simulink model "AcermanDynExt"  (R2021a)
settings: Solver=FixedStepAuto  StartTime=0.0  StopTime=simTime  RelTol=1e-3
values from neighbouring files (symbols this model uses):
  a = 2    [Ackerman_init.m]
  a0 = 1    [Ackerman_init.m]
  a1 = 4    [Ackerman_init.m]
  a2 = 3    [Ackerman_init.m]
  b = 1.05*a    (= 2.1)    [Ackerman_init.m]
  Change = 0    [Ackerman_init.m]
  k0 = 1    [Ackerman_init.m]
  k1 = place(Ad,bd,pd)    [Ackerman_init.m]
  k2 = place(Ac,bc,lambdatr')    [Ackerman_init.m]
  l = ylabel('$\omega(t)$' )    [Ackerman_init.m]
  pathType = 1    [Ackerman_init.m]
  phi0 = 0    [Ackerman_init.m]
  r = 2    [Ackerman_init.m]
  ref0 = [0 0]'    [Ackerman_init.m]
  refType = 1    [Ackerman_init.m]
  T = 0.1    [Ackerman_init.m]
  theta0 = pi/2    (= 1.57079632679)    [Ackerman_init.m]
  v0 = 1    [Ackerman_init.m]
  v_ref = 2    [Ackerman_init.m]
  x0 = 1    [Ackerman_init.m]
  y0 = 1    [Ackerman_init.m]
libraries: robotmobilelib x5
(part 1 of 4)
settings Model: Creator=mohd-  LastModifiedBy=mebbaid
settings SolverCC: AlgebraicLoopSolver=TrustRegion
settings DebuggingCC: SFMachineParentedDataDiag=warning

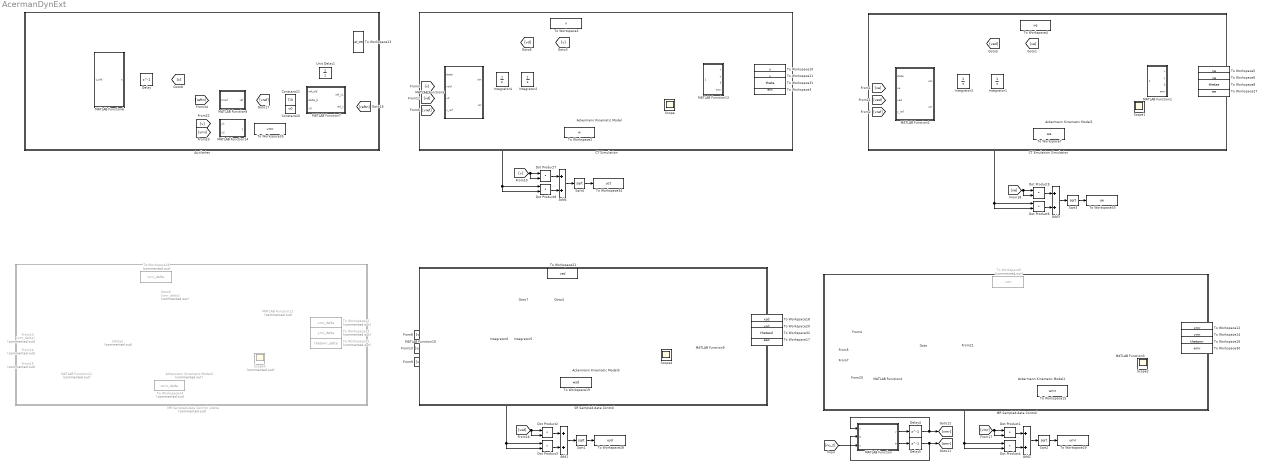
== system AcermanDynExt ==
  Ackermann Kinematic Model{,1..3} (4 alike) : robotmobilelib/Ackermann Kinematic Model  WheelBase=l  VehicleSpeedRange=[-inf inf]  MaxSteeringAngle=pi/3  InitialState=[x0; y0; theta0; phi0]  SimulateUsing=Interpreted execution
      settings: SourceProductBaseCode=RO
  Ackermann Kinematic Model4 : robotmobilelib/Ackermann Kinematic Model  Commented=on  WheelBase=l  VehicleSpeedRange=[-inf inf]  MaxSteeringAngle=pi/3  InitialState=[x0; y0; theta0; phi0]  SimulateUsing=Interpreted execution
      settings: SourceProductBaseCode=RO
  Add{1..4} (4 alike) : Sum
  Auxilaries : Subsystem
  CT Emulation Simulation : Subsystem
  CT Simulation : Subsystem
  Constant20 : Constant  Value=v0
  Constant21 : Constant  Value=T/3
  Delay : Delay  DelayLength=1  InitialCondition=0  SampleTime=T
  Delay2 : Delay  Commented=on  DelayLength=1  InitialCondition=v0  SampleTime=T
  Delay4 : Delay  DelayLength=1  InitialCondition=v0  SampleTime=T
  Delay5 : Delay  DelayLength=1  InitialCondition=0  SampleTime=T
  Dot Product{1..8} (8 alike) : DotProduct  InputSameDT=on  OutDataTypeStr=Inherit: Inherit via internal rule
  From10 : From  Commented=on  GotoTag=vmr_delta
  From14 : From  Commented=on  GotoTag=vref
  From15 : From  Commented=on  GotoTag=c
  Goto9 : Goto  Commented=on  GotoTag=vmr_delta
  Integrator1 : Integrator  InitialCondition=v0
  Integrator2 : Integrator  InitialCondition=v0
  Integrator3 : Integrator
  Integrator4 : Integrator
  Integrator5 : Integrator  InitialCondition=v0
  Integrator6 : Integrator
  MATLAB Function : MATLAB Function  TreatAsAtomicUnit=on  SystemSampleTime=T
  MATLAB Function1 : MATLAB Function  TreatAsAtomicUnit=on
  MATLAB Function10 : MATLAB Function  TreatAsAtomicUnit=on  SystemSampleTime=T
  MATLAB Function11 : MATLAB Function  Commented=on  TreatAsAtomicUnit=on
  MATLAB Function12 : MATLAB Function  Commented=on  TreatAsAtomicUnit=on  SystemSampleTime=T
  MATLAB Function13 : MATLAB Function  TreatAsAtomicUnit=on
  MATLAB Function14 : MATLAB Function  TreatAsAtomicUnit=on  SystemSampleTime=T
  MATLAB Function2 : MATLAB Function  TreatAsAtomicUnit=on  SystemSampleTime=T
  MATLAB Function3 : MATLAB Function  TreatAsAtomicUnit=on
  MATLAB Function4 : MATLAB Function  TreatAsAtomicUnit=on  SystemSampleTime=T/3
  MATLAB Function5 : MATLAB Function  TreatAsAtomicUnit=on
  MATLAB Function6 : MATLAB Function  TreatAsAtomicUnit=on  SystemSampleTime=T/3
  MATLAB Function7 : MATLAB Function  TreatAsAtomicUnit=on  SystemSampleTime=T
  MATLAB Function8 : MATLAB Function  TreatAsAtomicUnit=on
  MATLAB Function9 : MATLAB Function  TreatAsAtomicUnit=on
  MR Sampled-data Control : Subsystem
  MR Sampled-data Control ydelta : Subsystem  Commented=on
  SR Sampled-data Control : Subsystem
  Scope{,1..2,4} (4 alike) : Scope
  Scope3 : Scope  Commented=on
  Sqrt{1..4} (4 alike) : Sqrt  SaturateOnIntegerOverflow=on
  To Workspace1 : ToWorkspace  VariableName=v  SampleTime=10^-3
      settings: Save2DSignal=2-D array (concatenate along first dimension)
  To Workspace10 : ToWorkspace  VariableName=x  SampleTime=10^-3
      settings: Save2DSignal=2-D array (concatenate along first dimension)
  To Workspace11 : ToWorkspace  VariableName=y  SampleTime=10^-3
      settings: Save2DSignal=2-D array (concatenate along first dimension)
  To Workspace12 : ToWorkspace  VariableName=xmr  SampleTime=10^-3
      settings: Save2DSignal=2-D array (concatenate along first dimension)
  To Workspace13 : ToWorkspace  VariableName=ref_MR  SampleTime=T/3
  To Workspace14 : ToWorkspace  VariableName=ymr  SampleTime=10^-3
      settings: Save2DSignal=2-D array (concatenate along first dimension)
  To Workspace15 : ToWorkspace  VariableName=wmr  SampleTime=10^-3
      settings: Save2DSignal=2-D array (concatenate along first dimension)
  To Workspace16 : ToWorkspace  VariableName=thetamr  SampleTime=10^-3
      settings: Save2DSignal=2-D array (concatenate along first dimension)
  To Workspace17 : ToWorkspace  VariableName=esd  SampleTime=10^-3
      settings: Save2DSignal=2-D array (concatenate along first dimension)
  To Workspace18 : ToWorkspace  VariableName=xsd  SampleTime=10^-3
      settings: Save2DSignal=2-D array (concatenate along first dimension)
  To Workspace19 : ToWorkspace  VariableName=wsd  SampleTime=10^-3
      settings: Save2DSignal=2-D array (concatenate along first dimension)
  To Workspace2 : ToWorkspace  VariableName=w  SampleTime=10^-3
      settings: Save2DSignal=2-D array (concatenate along first dimension)
  To Workspace20 : ToWorkspace  VariableName=ysd  SampleTime=10^-3
      settings: Save2DSignal=2-D array (concatenate along first dimension)
  To Workspace21 : ToWorkspace  VariableName=vsd  SampleTime=10^-3
      settings: Save2DSignal=2-D array (concatenate along first dimension)
  To Workspace22 : ToWorkspace  Commented=on  VariableName=xmr_delta  SampleTime=10^-3
      settings: Save2DSignal=2-D array (concatenate along first dimension)
  To Workspace23 : ToWorkspace  Commented=on  VariableName=ymr_delta  SampleTime=10^-3
      settings: Save2DSignal=2-D array (concatenate along first dimension)
  To Workspace24 : ToWorkspace  Commented=on  VariableName=wmr_delta  SampleTime=10^-3
      settings: Save2DSignal=2-D array (concatenate along first dimension)
  To Workspace25 : ToWorkspace  Commented=on  VariableName=thetamr_delta  SampleTime=10^-3
      settings: Save2DSignal=2-D array (concatenate along first dimension)
  To Workspace26 : ToWorkspace  Commented=on  VariableName=vmr_delta  SampleTime=10^-3
      settings: Save2DSignal=2-D array (concatenate along first dimension)
  To Workspace27 : ToWorkspace  VariableName=ee  SampleTime=10^-3
      settings: Save2DSignal=2-D array (concatenate along first dimension)
  To Workspace28 : ToWorkspace  VariableName=usd  SampleTime=10^-3
      settings: Save2DSignal=2-D array (concatenate along first dimension)
  To Workspace29 : ToWorkspace  VariableName=umr  SampleTime=10^-3
      settings: Save2DSignal=2-D array (concatenate along first dimension)
  To Workspace3 : ToWorkspace  VariableName=ect  SampleTime=10^-3
      settings: Save2DSignal=2-D array (concatenate along first dimension)
  To Workspace30 : ToWorkspace  VariableName=emr  SampleTime=10^-3
      settings: Save2DSignal=2-D array (concatenate along first dimension)
  To Workspace31 : ToWorkspace  VariableName=theta  SampleTime=10^-3
      settings: Save2DSignal=2-D array (concatenate along first dimension)
  To Workspace32 : ToWorkspace  VariableName=thetasd  SampleTime=10^-3
      settings: Save2DSignal=2-D array (concatenate along first dimension)
  To Workspace33 : ToWorkspace  VariableName=ue  SampleTime=10^-3
      settings: Save2DSignal=2-D array (concatenate along first dimension)
  To Workspace34 : ToWorkspace  VariableName=uct  SampleTime=10^-3
      settings: Save2DSignal=2-D array (concatenate along first dimension)
  To Workspace35 : ToWorkspace  VariableName=vmr  SampleTime=10^-3
      settings: Save2DSignal=2-D array (concatenate along first dimension)
  To Workspace4 : ToWorkspace  VariableName=ve  SampleTime=10^-3
      settings: Save2DSignal=2-D array (concatenate along first dimension)
  To Workspace5 : ToWorkspace  VariableName=xe  SampleTime=10^-3
      settings: Save2DSignal=2-D array (concatenate along first dimension)
  To Workspace6 : ToWorkspace  VariableName=ye  SampleTime=10^-3
      settings: Save2DSignal=2-D array (concatenate along first dimension)
  To Workspace7 : ToWorkspace  VariableName=we  SampleTime=10^-3
      settings: Save2DSignal=2-D array (concatenate along first dimension)
  To Workspace8 : ToWorkspace  VariableName=thetae  SampleTime=10^-3
      settings: Save2DSignal=2-D array (concatenate along first dimension)
  To Workspace9 : ToWorkspace  Commented=on  VariableName=vmr  SampleTime=10^-3
      settings: Save2DSignal=2-D array (concatenate along first dimension)
  Unit Delay1 : UnitDelay  InitialCondition=ref0  SampleTime=T/3  HasFrameUpgradeWarning=on
  wires:
  Ackermann Kinematic Model3/2 -> Scope4/1
  Ackermann Kinematic Model2/1 -> MATLAB Function4/1(state), MATLAB Function3/1(state)
  [vmr] -> MATLAB Function4/2(v)
  Constant20/1 -> MATLAB Function7/3(v0)
  Ackermann Kinematic Model2/2 -> Scope2/1
  MATLAB Function1/1(x) -> To Workspace5/1
  Delay/1 -> [c], MATLAB Function6/1(c_old)
  MATLAB Function1/3(theta) -> To Workspace8/1
  MATLAB Function10/2(utr) -> Dot Product3/2, Dot Product3/1, To Workspace19/1, Ackermann Kinematic Model3/2
  MATLAB Function5/1(utn) -> Integrator4/1
  [vref] -> MATLAB Function10/4(v_ref)
  MATLAB Function6/1(c) -> Delay/1
  [c] -> MATLAB Function4/4(c)
  MATLAB Function8/1(ref) -> [vref]
  [v] -> MATLAB Function5/2(vold)
  Ackermann Kinematic Model/2 -> Scope/1
  [vref] -> MATLAB Function5/4(v_ref)
  MATLAB Function2/1(utn) -> Integrator3/1
  Integrator2/1 -> To Workspace1/1, [v], Ackermann Kinematic Model/1
  [ve] -> MATLAB Function2/2(ve)
  Ackermann Kinematic Model1/2 -> Scope1/1
  MATLAB Function7/1(ref_x1) -> To Workspace13/1, Unit Delay1/1
  [vref] -> MATLAB Function2/4(v_ref)
  Ackermann Kinematic Model1/1 -> MATLAB Function2/1(state), MATLAB Function1/1(state)
  MATLAB Function1/2(y) -> To Workspace6/1
  [vsd] -> MATLAB Function10/2(v)
  MATLAB Function7/2(ref_x) -> [reftn]
  [vref] -> MATLAB Function4/3(v_ref)
  [reftn] -> MATLAB Function8/1(tnref)
  Integrator1/1 -> To Workspace4/1, [ve], Ackermann Kinematic Model1/1
  Constant21/1 -> MATLAB Function7/2(delta_b)
  MATLAB Function10/1(utn) -> Integrator6/1
  Integrator5/1 -> To Workspace21/1, [vsd], Ackermann Kinematic Model3/1
  Unit Delay1/1 -> MATLAB Function7/1(ref_old)
  Integrator3/1 -> [ved], Integrator1/1
  [ved] -> MATLAB Function2/3(ved)
  Integrator4/1 -> [vd], Integrator2/1
  [vd] -> MATLAB Function5/3(vd)
  Integrator6/1 -> [vsdd], Integrator5/1
  [vsdd] -> MATLAB Function10/3(vsdd)
  MATLAB Function11/1(x) -> To Workspace22/1
  MATLAB Function12/2(w) -> To Workspace24/1, Ackermann Kinematic Model4/2
  MATLAB Function11/2(y) -> To Workspace23/1
  Ackermann Kinematic Model4/2 -> Scope3/1
  Delay2/1 -> To Workspace26/1, Goto9/1, Ackermann Kinematic Model4/1
  From14/1 -> MATLAB Function12/3(v_ref)
  MATLAB Function12/1(u) -> Delay2/1
  From15/1 -> MATLAB Function12/4(c)
  MATLAB Function11/3(theta) -> To Workspace25/1
  Ackermann Kinematic Model4/1 -> MATLAB Function12/1(state), MATLAB Function11/1(state)
  From10/1 -> MATLAB Function12/2(v)
  MATLAB Function3/2(y) -> To Workspace14/1
  MATLAB Function3/1(x) -> To Workspace12/1
  MATLAB Function3/3(theta) -> To Workspace16/1
  MATLAB Function3/4(emr) -> To Workspace30/1
  MATLAB Function1/4(emr) -> To Workspace27/1
  Ackermann Kinematic Model/1 -> MATLAB Function13/1(state), MATLAB Function5/1(state)
  MATLAB Function13/3(theta) -> To Workspace31/1
  MATLAB Function13/4(emr) -> To Workspace3/1
  MATLAB Function13/1(x) -> To Workspace10/1
  MATLAB Function13/2(y) -> To Workspace11/1
  Ackermann Kinematic Model3/1 -> MATLAB Function9/1(state), MATLAB Function10/1(state)
  MATLAB Function9/3(theta) -> To Workspace32/1
  MATLAB Function9/4(emr) -> To Workspace17/1
  MATLAB Function9/1(x) -> To Workspace18/1
  MATLAB Function9/2(y) -> To Workspace20/1
  Add1/1 -> Sqrt1/1
  Dot Product2/1 -> Add1/1
  Dot Product3/1 -> Add1/2
  Sqrt1/1 -> To Workspace28/1
  [vsd] -> Dot Product2/2, Dot Product2/1
  Dot Product1/1 -> Add2/1
  Dot Product4/1 -> Add2/2
  Sqrt2/1 -> To Workspace29/1
  Add2/1 -> Sqrt2/1
  MATLAB Function4/2(w) -> Dot Product4/1, Dot Product4/2, To Workspace15/1, Ackermann Kinematic Model2/2
  [vmr] -> Dot Product1/2, Dot Product1/1
  Dot Product5/1 -> Add3/1
  Dot Product6/1 -> Add3/2
  Sqrt3/1 -> To Workspace33/1
  Add3/1 -> Sqrt3/1
  MATLAB Function2/2(utr) -> Dot Product6/1, Dot Product6/2, To Workspace7/1, Ackermann Kinematic Model1/2
  [ve] -> Dot Product5/2, Dot Product5/1
  Dot Product7/1 -> Add4/1
  Dot Product8/1 -> Add4/2
  Sqrt4/1 -> To Workspace34/1
  Add4/1 -> Sqrt4/1
  MATLAB Function5/2(utr) -> Dot Product8/1, Dot Product8/2, To Workspace2/1, Ackermann Kinematic Model/2
  [v] -> Dot Product7/2, Dot Product7/1
  [vmr] -> To Workspace9/1, Ackermann Kinematic Model2/1
  [amr] -> MATLAB Function4/5(amr)
  MATLAB Function/1(v) -> Delay4/1
  MATLAB Function/2(a) -> Delay5/1
  Delay4/1 -> MATLAB Function/1("v "), [vmr]
  Delay5/1 -> [amr], MATLAB Function/2("a ")
  MATLAB Function4/1(u) -> [nu_2]
  [nu_2] -> MATLAB Function/3(u)
  [v] -> MATLAB Function14/1(u1)
  MATLAB Function14/1(y) -> To Workspace35/1
  [vmr] -> MATLAB Function14/2(u2)

== system AcermanDynExt/Auxilaries ==

== system AcermanDynExt/CT Emulation Simulation ==

== system AcermanDynExt/CT Simulation ==

== system AcermanDynExt/MR Sampled-data Control ==

== system AcermanDynExt/MR Sampled-data Control ydelta ==

== system AcermanDynExt/SR Sampled-data Control ==

== matlab function AcermanDynExt/MATLAB Function4 ==
  data: state input; v input; v_ref input; c input; amr input; pathType parameter; r parameter; a2 parameter; a1 parameter; a0 parameter; k0 parameter; l parameter; u output; w output; Change parameter; T parameter; refType parameter
function [u,w] = MATLAB_Function5(state, v, v_ref, c , amr,pathType, r, a2, a1, a0, k0, l , Change, T, refType)

x = state(1); y = state(2); z = state(3); theta = state(4);

d = T/3; 
if refType == 1
    lamda1 = k0; lamda2 = k0;
    L0 = -(exp(-T*lamda1) + exp(-T*lamda2) - exp(-T*lamda1)*exp(-T*lamda2) - 1)/T^2;
    L1 = -(exp(-T*lamda1) + exp(-T*lamda2) + exp(-T*lamda1)*exp(-T*lamda2) - 3)/(2*T);
else
    L0 = 0;
    L1 = 0;
end
 

if pathType == 1
    w0 = [   -(2*a2*l^2*v^2*cos(theta)^2 - 2*v^3*y*sin(z) - a0*l^2*r^2*cos(theta)^2 - 2*v^3*x*cos(z) + a0*l^2*x^2*cos(theta)^2 + a0*l^2*y^2*cos(theta)^2 + 2*v^3*x*cos(theta)^2*cos(z) + 2*v^3*y*cos(theta)^2*sin(z) + 2*a1*l^2*v*x*cos(theta)^2*cos(z) + 2*a1*l^2*v*y*cos(theta)^2*sin(z) + 2*a2*l*v^2*y*cos(theta)*cos(z)*sin(theta) - 2*a2*l*v^2*x*cos(theta)*sin(theta)*sin(z))/(2*l*v^2*(y*cos(z) - x*sin(z)));
             -(2*a2*l^2*v^2*cos(theta)^2 - 2*v^3*y*sin(z) - a0*l^2*r^2*cos(theta)^2 - 2*v^3*x*cos(z) + a0*l^2*x^2*cos(theta)^2 + a0*l^2*y^2*cos(theta)^2 + 2*v^3*x*cos(theta)^2*cos(z) + 2*v^3*y*cos(theta)^2*sin(z) + 2*a1*l^2*v*x*cos(theta)^2*cos(z) + 2*a1*l^2*v*y*cos(theta)^2*sin(z) + 2*a2*l*v^2*y*cos(theta)*cos(z)*sin(theta) - 2*a2*l*v^2*x*cos(theta)*sin(theta)*sin(z))/(2*l*v^2*(y*cos(z) - x*sin(z)));
             -(2*a2*l^2*v^2*cos(theta)^2 - 2*v^3*y*sin(z) - a0*l^2*r^2*cos(theta)^2 - 2*v^3*x*cos(z) + a0*l^2*x^2*cos(theta)^2 + a0*l^2*y^2*cos(theta)^2 + 2*v^3*x*cos(theta)^2*cos(z) + 2*v^3*y*cos(theta)^2*sin(z) + 2*a1*l^2*v*x*cos(theta)^2*cos(z) + 2*a1*l^2*v*y*cos(theta)^2*sin(z) + 2*a2*l*v^2*y*cos(theta)*cos(z)*sin(theta) - 2*a2*l*v^2*x*cos(theta)*sin(theta)*sin(z))/(2*l*v^2*(y*cos(z) - x*sin(z)))]; 
 
    w1 = [  -(3*(2*l*v^6*y*cos(theta)^3*cos(z) - 2*v^6*y^2*cos(z)^2*sin(theta) - 2*v^6*x^2*sin(theta)*sin(z)^2 - 2*v^6*y^2*sin(theta)*sin(z)^2 - 2*v^6*x^2*cos(z)^2*sin(theta) - 2*l*v^6*x*cos(theta)^3*sin(z) - 2*v^6*x^2*cos(theta)^2*cos(z)^2*sin(theta) + 4*v^6*x^2*cos(theta)^4*cos(z)^2*sin(theta) + 2*v^6*y^2*cos(theta)^2*cos(z)^2*sin(theta) + 2*v^6*x^2*cos(theta)^2*sin(theta)*sin(z)^2 - 2*v^6*y^2*cos(theta)^2*sin(theta)*sin(z)^2 + 4*v^6*y^2*cos(theta)^4*sin(theta)*sin(z)^2 - 2*l*v^6*y*cos(theta)*cos(z) + a0^2*l^4*r^4*cos(theta)^4*sin(theta) + 2*l*v^6*x*cos(theta)*sin(z) + 4*a2^2*l^4*v^4*cos(theta)^4*sin(theta) + a0^2*l^4*x^4*cos(theta)^4*sin(theta) + a0^2*l^4*y^4*cos(theta)^4*sin(theta) - 2*a2^2*l^3*v^4*y*cos(theta)^3*cos(z) + 2*a2^2*l^3*v^4*x*cos(theta)^3*sin(z) - 2*a0^2*l^4*r^2*x^2*cos(theta)^4*sin(theta) - 2*a0^2*l^4*r^2*y^2*cos(theta)^4*sin(theta) + 2*a0^2*l^4*x^2*y^2*cos(theta)^4*sin(theta) + 2*a1*l^3*v^4*y*cos(theta)^3*cos(z) - 2*a1*l^3*v^4*x*cos(theta)^3*sin(z) - 2*a2^2*l^2*v^4*x^2*cos(theta)^2*sin(theta)*sin(z)^2 + 4*a1^2*l^4*v^2*y^2*cos(theta)^4*sin(theta)*sin(z)^2 - 8*v^6*x*y*cos(theta)^2*cos(z)*sin(theta)*sin(z) + 8*v^6*x*y*cos(theta)^4*cos(z)*sin(theta)*sin(z) - a0*l^2*v^3*x^3*cos(theta)^2*cos(z)*sin(theta) + 4*a0*l^2*v^3*x^3*cos(theta)^4*cos(z)*sin(theta) - 2*a0*l^3*v^3*x^2*cos(theta)^3*cos(z)*sin(z) + 2*a0*l^3*v^3*y^2*cos(theta)^3*cos(z)*sin(z) - a0*l^2*v^3*y^3*cos(theta)^2*sin(theta)*sin(z) + 4*a0*l^2*v^3*y^3*cos(theta)^4*sin(theta)*sin(z) + 4*a2^2*l^2*v^4*y^2*cos(theta)^2*cos(z)^2*sin(theta)^3 + 4*a2^2*l^2*v^4*x^2*cos(theta)^2*sin(theta)^3*sin(z)^2 - 2*a1*l^2*v^4*x^2*cos(theta)^2*cos(z)^2*sin(theta) + 8*a1*l^2*v^4*x^2*cos(theta)^4*cos(z)^2*sin(theta) + 2*a1*l^2*v^4*y^2*cos(theta)^2*cos(z)^2*sin(theta) + 8*a2^2*l^3*v^4*y*cos(theta)^3*cos(z)*sin(theta)^2 + 2*a1*l^2*v^4*x^2*cos(theta)^2*sin(theta)*sin(z)^2 - 8*a2^2*l^3*v^4*x*cos(theta)^3*sin(theta)^2*sin(z) - 2*a1*l^2*v^4*y^2*cos(theta)^2*sin(theta)*sin(z)^2 + 8*a1*l^2*v^4*y^2*cos(theta)^4*sin(theta)*sin(z)^2 - a0*a2*l^3*v^2*y^3*cos(theta)^3*cos(z) - 4*a0*a2*l^4*r^2*v^2*cos(theta)^4*sin(theta) + 4*a0*a2*l^4*v^2*x^2*cos(theta)^4*sin(theta) + 4*a0*a2*l^4*v^2*y^2*cos(theta)^4*sin(theta) + a0*a2*l^3*v^2*x^3*cos(theta)^3*sin(z) + 2*a0*l^3*v^3*x*y*cos(theta)^3*cos(z)^2 - 2*a2*l^2*v^5*x*cos(theta)^2*cos(z)*sin(theta) + 8*a2*l^2*v^5*x*cos(theta)^4*cos(z)*sin(theta) - 2*a0*l^3*v^3*x*y*cos(theta)^3*sin(z)^2 - 2*a2*l^2*v^5*y*cos(theta)^2*sin(theta)*sin(z) + 8*a2*l^2*v^5*y*cos(theta)^4*sin(theta)*sin(z) + 4*a1^2*l^4*v^2*x^2*cos(theta)^4*cos(z)^2*sin(theta) - 2*a2^2*l^2*v^4*y^2*cos(theta)^2*cos(z)^2*sin(theta) - 4*a0*a2*l^3*v^2*x^3*cos(theta)^3*sin(theta)^2*sin(z) + a0*a2*l^3*r^2*v^2*y*cos(theta)^3*cos(z) - 8*a2*l*v^5*x^2*cos(theta)^3*cos(z)*sin(theta)^2*sin(z) + 8*a2*l*v^5*y^2*cos(theta)^3*cos(z)*sin(theta)^2*sin(z) - a0*a2*l^3*v^2*x^2*y*cos(theta)^3*cos(z) - 2*a1*a2*l^3*v^3*x*y*cos(theta)^3*cos(z)^2 - a0*a2*l^3*r^2*v^2*x*cos(theta)^3*sin(z) + 4*a0*a1*l^4*v*x^3*cos(theta)^4*cos(z)*sin(theta) + 8*a1*a2*l^4*v^3*x*cos(theta)^4*cos(z)*sin(theta) + a0*a2*l^3*v^2*x*y^2*cos(theta)^3*sin(z) + 2*a1*a2*l^3*v^3*x*y*cos(theta)^3*sin(z)^2 + 4*a0*a1*l^4*v*y^3*cos(theta)^4*sin(theta)*sin(z) + 8*a1*a2*l^4*v^3*y*cos(theta)^4*sin(theta)*sin(z) - 2*a2*l*v^5*x*y*cos(theta)*cos(z)^2*sin(theta)^2 + 2*a2*l*v^5*x*y*cos(theta)*sin(theta)^2*sin(z)^2 + 2*a1*a2*l^3*v^3*x^2*cos(theta)^3*cos(z)*sin(z) - 2*a1*a2*l^3*v^3*y^2*cos(theta)^3*cos(z)*sin(z) + a0*l^2*r^2*v^3*x*cos(theta)^2*cos(z)*sin(theta) - 4*a0*l^2*r^2*v^3*x*cos(theta)^4*cos(z)*sin(theta) - a0*l^2*v^3*x*y^2*cos(theta)^2*cos(z)*sin(theta) + 4*a0*l^2*v^3*x*y^2*cos(theta)^4*cos(z)*sin(theta) + 8*a2*l*v^5*x*y*cos(theta)^3*cos(z)^2*sin(theta)^2 + a0*l^2*r^2*v^3*y*cos(theta)^2*sin(theta)*sin(z) - 4*a0*l^2*r^2*v^3*y*cos(theta)^4*sin(theta)*sin(z) - a0*l^2*v^3*x^2*y*cos(theta)^2*sin(theta)*sin(z) + 4*a0*l^2*v^3*x^2*y*cos(theta)^4*sin(theta)*sin(z) - 8*a2*l*v^5*x*y*cos(theta)^3*sin(theta)^2*sin(z)^2 + 2*a2*l*v^5*x^2*cos(theta)*cos(z)*sin(theta)^2*sin(z) - 2*a2*l*v^5*y^2*cos(theta)*cos(z)*sin(theta)^2*sin(z) + 4*a0*a2*l^3*v^2*y^3*cos(theta)^3*cos(z)*sin(theta)^2 - 8*a1*l^2*v^4*x*y*cos(theta)^2*cos(z)*sin(theta)*sin(z) + 16*a1*l^2*v^4*x*y*cos(theta)^4*cos(z)*sin(theta)*sin(z) - 4*a0*a2*l^3*r^2*v^2*y*cos(theta)^3*cos(z)*sin(theta)^2 + 4*a0*a2*l^3*v^2*x^2*y*cos(theta)^3*cos(z)*sin(theta)^2 + 8*a1*a2*l^3*v^3*x*y*cos(theta)^3*cos(z)^2*sin(theta)^2 + 4*a0*a2*l^3*r^2*v^2*x*cos(theta)^3*sin(theta)^2*sin(z) - 4*a0*a2*l^3*v^2*x*y^2*cos(theta)^3*sin(theta)^2*sin(z) - 8*a1*a2*l^3*v^3*x*y*cos(theta)^3*sin(theta)^2*sin(z)^2 + 4*a2^2*l^2*v^4*x*y*cos(theta)^2*cos(z)*sin(theta)*sin(z) + 8*a1^2*l^4*v^2*x*y*cos(theta)^4*cos(z)*sin(theta)*sin(z) - 4*a0*a1*l^4*r^2*v*x*cos(theta)^4*cos(z)*sin(theta) + 4*a0*a1*l^4*v*x*y^2*cos(theta)^4*cos(z)*sin(theta) - 4*a0*a1*l^4*r^2*v*y*cos(theta)^4*sin(theta)*sin(z) + 4*a0*a1*l^4*v*x^2*y*cos(theta)^4*sin(theta)*sin(z) - 8*a1*a2*l^3*v^3*x^2*cos(theta)^3*cos(z)*sin(theta)^2*sin(z) + 8*a1*a2*l^3*v^3*y^2*cos(theta)^3*cos(z)*sin(theta)^2*sin(z) - 8*a2^2*l^2*v^4*x*y*cos(theta)^2*cos(z)*sin(theta)^3*sin(z)))/(8*l^2*v^4*cos(theta)*(y*cos(z) - x*sin(z))^2);
            -(3*(2*l*v^6*y*cos(theta)^3*cos(z) - 2*v^6*y^2*cos(z)^2*sin(theta) - 2*v^6*x^2*sin(theta)*sin(z)^2 - 2*v^6*y^2*sin(theta)*sin(z)^2 - 2*v^6*x^2*cos(z)^2*sin(theta) - 2*l*v^6*x*cos(theta)^3*sin(z) - 2*v^6*x^2*cos(theta)^2*cos(z)^2*sin(theta) + 4*v^6*x^2*cos(theta)^4*cos(z)^2*sin(theta) + 2*v^6*y^2*cos(theta)^2*cos(z)^2*sin(theta) + 2*v^6*x^2*cos(theta)^2*sin(theta)*sin(z)^2 - 2*v^6*y^2*cos(theta)^2*sin(theta)*sin(z)^2 + 4*v^6*y^2*cos(theta)^4*sin(theta)*sin(z)^2 - 2*l*v^6*y*cos(theta)*cos(z) + a0^2*l^4*r^4*cos(theta)^4*sin(theta) + 2*l*v^6*x*cos(theta)*sin(z) + 4*a2^2*l^4*v^4*cos(theta)^4*sin(theta) + a0^2*l^4*x^4*cos(theta)^4*sin(theta) + a0^2*l^4*y^4*cos(theta)^4*sin(theta) - 2*a2^2*l^3*v^4*y*cos(theta)^3*cos(z) + 2*a2^2*l^3*v^4*x*cos(theta)^3*sin(z) - 2*a0^2*l^4*r^2*x^2*cos(theta)^4*sin(theta) - 2*a0^2*l^4*r^2*y^2*cos(theta)^4*sin(theta) + 2*a0^2*l^4*x^2*y^2*cos(theta)^4*sin(theta) + 2*a1*l^3*v^4*y*cos(theta)^3*cos(z) - 2*a1*l^3*v^4*x*cos(theta)^3*sin(z) - 2*a2^2*l^2*v^4*x^2*cos(theta)^2*sin(theta)*sin(z)^2 + 4*a1^2*l^4*v^2*y^2*cos(theta)^4*sin(theta)*sin(z)^2 - 8*v^6*x*y*cos(theta)^2*cos(z)*sin(theta)*sin(z) + 8*v^6*x*y*cos(theta)^4*cos(z)*sin(theta)*sin(z) - a0*l^2*v^3*x^3*cos(theta)^2*cos(z)*sin(theta) + 4*a0*l^2*v^3*x^3*cos(theta)^4*cos(z)*sin(theta) - 2*a0*l^3*v^3*x^2*cos(theta)^3*cos(z)*sin(z) + 2*a0*l^3*v^3*y^2*cos(theta)^3*cos(z)*sin(z) - a0*l^2*v^3*y^3*cos(theta)^2*sin(theta)*sin(z) + 4*a0*l^2*v^3*y^3*cos(theta)^4*sin(theta)*sin(z) + 4*a2^2*l^2*v^4*y^2*cos(theta)^2*cos(z)^2*sin(theta)^3 + 4*a2^2*l^2*v^4*x^2*cos(theta)^2*sin(theta)^3*sin(z)^2 - 2*a1*l^2*v^4*x^2*cos(theta)^2*cos(z)^2*sin(theta) + 8*a1*l^2*v^4*x^2*cos(theta)^4*cos(z)^2*sin(theta) + 2*a1*l^2*v^4*y^2*cos(theta)^2*cos(z)^2*sin(theta) + 8*a2^2*l^3*v^4*y*cos(theta)^3*cos(z)*sin(theta)^2 + 2*a1*l^2*v^4*x^2*cos(theta)^2*sin(theta)*sin(z)^2 - 8*a2^2*l^3*v^4*x*cos(theta)^3*sin(theta)^2*sin(z) - 2*a1*l^2*v^4*y^2*cos(theta)^2*sin(theta)*sin(z)^2 + 8*a1*l^2*v^4*y^2*cos(theta)^4*sin(theta)*sin(z)^2 - a0*a2*l^3*v^2*y^3*cos(theta)^3*cos(z) - 4*a0*a2*l^4*r^2*v^2*cos(theta)^4*sin(theta) + 4*a0*a2*l^4*v^2*x^2*cos(theta)^4*sin(theta) + 4*a0*a2*l^4*v^2*y^2*cos(theta)^4*sin(theta) + a0*a2*l^3*v^2*x^3*cos(theta)^3*sin(z) + 2*a0*l^3*v^3*x*y*cos(theta)^3*cos(z)^2 - 2*a2*l^2*v^5*x*cos(theta)^2*cos(z)*sin(theta) + 8*a2*l^2*v^5*x*cos(theta)^4*cos(z)*sin(theta) - 2*a0*l^3*v^3*x*y*cos(theta)^3*sin(z)^2 - 2*a2*l^2*v^5*y*cos(theta)^2*sin(theta)*sin(z) + 8*a2*l^2*v^5*y*cos(theta)^4*sin(theta)*sin(z) + 4*a1^2*l^4*v^2*x^2*cos(theta)^4*cos(z)^2*sin(theta) - 2*a2^2*l^2*v^4*y^2*cos(theta)^2*cos(z)^2*sin(theta) - 4*a0*a2*l^3*v^2*x^3*cos(theta)^3*sin(theta)^2*sin(z) + a0*a2*l^3*r^2*v^2*y*cos(theta)^3*cos(z) - 8*a2*l*v^5*x^2*cos(theta)^3*cos(z)*sin(theta)^2*sin(z) + 8*a2*l*v^5*y^2*cos(theta)^3*cos(z)*sin(theta)^2*sin(z) - a0*a2*l^3*v^2*x^2*y*cos(theta)^3*cos(z) - 2*a1*a2*l^3*v^3*x*y*cos(theta)^3*cos(z)^2 - a0*a2*l^3*r^2*v^2*x*cos(theta)^3*sin(z) + 4*a0*a1*l^4*v*x^3*cos(theta)^4*cos(z)*sin(theta) + 8*a1*a2*l^4*v^3*x*cos(theta)^4*cos(z)*sin(theta) + a0*a2*l^3*v^2*x*y^2*cos(theta)^3*sin(z) + 2*a1*a2*l^3*v^3*x*y*cos(theta)^3*sin(z)^2 + 4*a0*a1*l^4*v*y^3*cos(theta)^4*sin(theta)*sin(z) + 8*a1*a2*l^4*v^3*y*cos(theta)^4*sin(theta)*sin(z) - 2*a2*l*v^5*x*y*cos(theta)*cos(z)^2*sin(theta)^2 + 2*a2*l*v^5*x*y*cos(theta)*sin(theta)^2*sin(z)^2 + 2*a1*a2*l^3*v^3*x^2*cos(theta)^3*cos(z)*sin(z) - 2*a1*a2*l^3*v^3*y^2*cos(theta)^3*cos(z)*sin(z) + a0*l^2*r^2*v^3*x*cos(theta)^2*cos(z)*sin(theta) - 4*a0*l^2*r^2*v^3*x*cos(theta)^4*cos(z)*sin(theta) - a0*l^2*v^3*x*y^2*cos(theta)^2*cos(z)*sin(theta) + 4*a0*l^2*v^3*x*y^2*cos(theta)^4*cos(z)*sin(theta) + 8*a2*l*v^5*x*y*cos(theta)^3*cos(z)^2*sin(theta)^2 + a0*l^2*r^2*v^3*y*cos(theta)^2*sin(theta)*sin(z) - 4*a0*l^2*r^2*v^3*y*cos(theta)^4*sin(theta)*sin(z) - a0*l^2*v^3*x^2*y*cos(theta)^2*sin(theta)*sin(z) + 4*a0*l^2*v^3*x^2*y*cos(theta)^4*sin(theta)*sin(z) - 8*a2*l*v^5*x*y*cos(theta)^3*sin(theta)^2*sin(z)^2 + 2*a2*l*v^5*x^2*cos(theta)*cos(z)*sin(theta)^2*sin(z) - 2*a2*l*v^5*y^2*cos(theta)*cos(z)*sin(theta)^2*sin(z) + 4*a0*a2*l^3*v^2*y^3*cos(theta)^3*cos(z)*sin(theta)^2 - 8*a1*l^2*v^4*x*y*cos(theta)^2*cos(z)*sin(theta)*sin(z) + 16*a1*l^2*v^4*x*y*cos(theta)^4*cos(z)*sin(theta)*sin(z) - 4*a0*a2*l^3*r^2*v^2*y*cos(theta)^3*cos(z)*sin(theta)^2 + 4*a0*a2*l^3*v^2*x^2*y*cos(theta)^3*cos(z)*sin(theta)^2 + 8*a1*a2*l^3*v^3*x*y*cos(theta)^3*cos(z)^2*sin(theta)^2 + 4*a0*a2*l^3*r^2*v^2*x*cos(theta)^3*sin(theta)^2*sin(z) - 4*a0*a2*l^3*v^2*x*y^2*cos(theta)^3*sin(theta)^2*sin(z) - 8*a1*a2*l^3*v^3*x*y*cos(theta)^3*sin(theta)^2*sin(z)^2 + 4*a2^2*l^2*v^4*x*y*cos(theta)^2*cos(z)*sin(theta)*sin(z) + 8*a1^2*l^4*v^2*x*y*cos(theta)^4*cos(z)*sin(theta)*sin(z) - 4*a0*a1*l^4*r^2*v*x*cos(theta)^4*cos(z)*sin(theta) + 4*a0*a1*l^4*v*x*y^2*cos(theta)^4*cos(z)*sin(theta) - 4*a0*a1*l^4*r^2*v*y*cos(theta)^4*sin(theta)*sin(z) + 4*a0*a1*l^4*v*x^2*y*cos(theta)^4*sin(theta)*sin(z) - 8*a1*a2*l^3*v^3*x^2*cos(theta)^3*cos(z)*sin(theta)^2*sin(z) + 8*a1*a2*l^3*v^3*y^2*cos(theta)^3*cos(z)*sin(theta)^2*sin(z) - 8*a2^2*l^2*v^4*x*y*cos(theta)^2*cos(z)*sin(theta)^3*sin(z)))/(2*l^2*v^4*cos(theta)*(y*cos(z) - x*sin(z))^2);
            -(21*(2*l*v^6*y*cos(theta)^3*cos(z) - 2*v^6*y^2*cos(z)^2*sin(theta) - 2*v^6*x^2*sin(theta)*sin(z)^2 - 2*v^6*y^2*sin(theta)*sin(z)^2 - 2*v^6*x^2*cos(z)^2*sin(theta) - 2*l*v^6*x*cos(theta)^3*sin(z) - 2*v^6*x^2*cos(theta)^2*cos(z)^2*sin(theta) + 4*v^6*x^2*cos(theta)^4*cos(z)^2*sin(theta) + 2*v^6*y^2*cos(theta)^2*cos(z)^2*sin(theta) + 2*v^6*x^2*cos(theta)^2*sin(theta)*sin(z)^2 - 2*v^6*y^2*cos(theta)^2*sin(theta)*sin(z)^2 + 4*v^6*y^2*cos(theta)^4*sin(theta)*sin(z)^2 - 2*l*v^6*y*cos(theta)*cos(z) + a0^2*l^4*r^4*cos(theta)^4*sin(theta) + 2*l*v^6*x*cos(theta)*sin(z) + 4*a2^2*l^4*v^4*cos(theta)^4*sin(theta) + a0^2*l^4*x^4*cos(theta)^4*sin(theta) + a0^2*l^4*y^4*cos(theta)^4*sin(theta) - 2*a2^2*l^3*v^4*y*cos(theta)^3*cos(z) + 2*a2^2*l^3*v^4*x*cos(theta)^3*sin(z) - 2*a0^2*l^4*r^2*x^2*cos(theta)^4*sin(theta) - 2*a0^2*l^4*r^2*y^2*cos(theta)^4*sin(theta) + 2*a0^2*l^4*x^2*y^2*cos(theta)^4*sin(theta) + 2*a1*l^3*v^4*y*cos(theta)^3*cos(z) - 2*a1*l^3*v^4*x*cos(theta)^3*sin(z) - 2*a2^2*l^2*v^4*x^2*cos(theta)^2*sin(theta)*sin(z)^2 + 4*a1^2*l^4*v^2*y^2*cos(theta)^4*sin(theta)*sin(z)^2 - 8*v^6*x*y*cos(theta)^2*cos(z)*sin(theta)*sin(z) + 8*v^6*x*y*cos(theta)^4*cos(z)*sin(theta)*sin(z) - a0*l^2*v^3*x^3*cos(theta)^2*cos(z)*sin(theta) + 4*a0*l^2*v^3*x^3*cos(theta)^4*cos(z)*sin(theta) - 2*a0*l^3*v^3*x^2*cos(theta)^3*cos(z)*sin(z) + 2*a0*l^3*v^3*y^2*cos(theta)^3*cos(z)*sin(z) - a0*l^2*v^3*y^3*cos(theta)^2*sin(theta)*sin(z) + 4*a0*l^2*v^3*y^3*cos(theta)^4*sin(theta)*sin(z) + 4*a2^2*l^2*v^4*y^2*cos(theta)^2*cos(z)^2*sin(theta)^3 + 4*a2^2*l^2*v^4*x^2*cos(theta)^2*sin(theta)^3*sin(z)^2 - 2*a1*l^2*v^4*x^2*cos(theta)^2*cos(z)^2*sin(theta) + 8*a1*l^2*v^4*x^2*cos(theta)^4*cos(z)^2*sin(theta) + 2*a1*l^2*v^4*y^2*cos(theta)^2*cos(z)^2*sin(theta) + 8*a2^2*l^3*v^4*y*cos(theta)^3*cos(z)*sin(theta)^2 + 2*a1*l^2*v^4*x^2*cos(theta)^2*sin(theta)*sin(z)^2 - 8*a2^2*l^3*v^4*x*cos(theta)^3*sin(theta)^2*sin(z) - 2*a1*l^2*v^4*y^2*cos(theta)^2*sin(theta)*sin(z)^2 + 8*a1*l^2*v^4*y^2*cos(theta)^4*sin(theta)*sin(z)^2 - a0*a2*l^3*v^2*y^3*cos(theta)^3*cos(z) - 4*a0*a2*l^4*r^2*v^2*cos(theta)^4*sin(theta) + 4*a0*a2*l^4*v^2*x^2*cos(theta)^4*sin(theta) + 4*a0*a2*l^4*v^2*y^2*cos(theta)^4*sin(theta) + a0*a2*l^3*v^2*x^3*cos(theta)^3*sin(z) + 2*a0*l^3*v^3*x*y*cos(theta)^3*cos(z)^2 - 2*a2*l^2*v^5*x*cos(theta)^2*cos(z)*sin(theta) + 8*a2*l^2*v^5*x*cos(theta)^4*cos(z)*sin(theta) - 2*a0*l^3*v^3*x*y*cos(theta)^3*sin(z)^2 - 2*a2*l^2*v^5*y*cos(theta)^2*sin(theta)*sin(z) + 8*a2*l^2*v^5*y*cos(theta)^4*sin(theta)*sin(z) + 4*a1^2*l^4*v^2*x^2*cos(theta)^4*cos(z)^2*sin(theta) - 2*a2^2*l^2*v^4*y^2*cos(theta)^2*cos(z)^2*sin(theta) - 4*a0*a2*l^3*v^2*x^3*cos(theta)^3*sin(theta)^2*sin(z) + a0*a2*l^3*r^2*v^2*y*cos(theta)^3*cos(z) - 8*a2*l*v^5*x^2*cos(theta)^3*cos(z)*sin(theta)^2*sin(z) + 8*a2*l*v^5*y^2*cos(theta)^3*cos(z)*sin(theta)^2*sin(z) - a0*a2*l^3*v^2*x^2*y*cos(theta)^3*cos(z) - 2*a1*a2*l^3*v^3*x*y*cos(theta)^3*cos(z)^2 - a0*a2*l^3*r^2*v^2*x*cos(theta)^3*sin(z) + 4*a0*a1*l^4*v*x^3*cos(theta)^4*cos(z)*sin(theta) + 8*a1*a2*l^4*v^3*x*cos(theta)^4*cos(z)*sin(theta) + a0*a2*l^3*v^2*x*y^2*cos(theta)^3*sin(z) + 2*a1*a2*l^3*v^3*x*y*cos(theta)^3*sin(z)^2 + 4*a0*a1*l^4*v*y^3*cos(theta)^4*sin(theta)*sin(z) + 8*a1*a2*l^4*v^3*y*cos(theta)^4*sin(theta)*sin(z) - 2*a2*l*v^5*x*y*cos(theta)*cos(z)^2*sin(theta)^2 + 2*a2*l*v^5*x*y*cos(theta)*sin(theta)^2*sin(z)^2 + 2*a1*a2*l^3*v^3*x^2*cos(theta)^3*cos(z)*sin(z) - 2*a1*a2*l^3*v^3*y^2*cos(theta)^3*cos(z)*sin(z) + a0*l^2*r^2*v^3*x*cos(theta)^2*cos(z)*sin(theta) - 4*a0*l^2*r^2*v^3*x*cos(theta)^4*cos(z)*sin(theta) - a0*l^2*v^3*x*y^2*cos(theta)^2*cos(z)*sin(theta) + 4*a0*l^2*v^3*x*y^2*cos(theta)^4*cos(z)*sin(theta) + 8*a2*l*v^5*x*y*cos(theta)^3*cos(z)^2*sin(theta)^2 + a0*l^2*r^2*v^3*y*cos(theta)^2*sin(theta)*sin(z) - 4*a0*l^2*r^2*v^3*y*cos(theta)^4*sin(theta)*sin(z) - a0*l^2*v^3*x^2*y*cos(theta)^2*sin(theta)*sin(z) + 4*a0*l^2*v^3*x^2*y*cos(theta)^4*sin(theta)*sin(z) - 8*a2*l*v^5*x*y*cos(theta)^3*sin(theta)^2*sin(z)^2 + 2*a2*l*v^5*x^2*cos(theta)*cos(z)*sin(theta)^2*sin(z) - 2*a2*l*v^5*y^2*cos(theta)*cos(z)*sin(theta)^2*sin(z) + 4*a0*a2*l^3*v^2*y^3*cos(theta)^3*cos(z)*sin(theta)^2 - 8*a1*l^2*v^4*x*y*cos(theta)^2*cos(z)*sin(theta)*sin(z) + 16*a1*l^2*v^4*x*y*cos(theta)^4*cos(z)*sin(theta)*sin(z) - 4*a0*a2*l^3*r^2*v^2*y*cos(theta)^3*cos(z)*sin(theta)^2 + 4*a0*a2*l^3*v^2*x^2*y*cos(theta)^3*cos(z)*sin(theta)^2 + 8*a1*a2*l^3*v^3*x*y*cos(theta)^3*cos(z)^2*sin(theta)^2 + 4*a0*a2*l^3*r^2*v^2*x*cos(theta)^3*sin(theta)^2*sin(z) - 4*a0*a2*l^3*v^2*x*y^2*cos(theta)^3*sin(theta)^2*sin(z) - 8*a1*a2*l^3*v^3*x*y*cos(theta)^3*sin(theta)^2*sin(z)^2 + 4*a2^2*l^2*v^4*x*y*cos(theta)^2*cos(z)*sin(theta)*sin(z) + 8*a1^2*l^4*v^2*x*y*cos(theta)^4*cos(z)*sin(theta)*sin(z) - 4*a0*a1*l^4*r^2*v*x*cos(theta)^4*cos(z)*sin(theta) + 4*a0*a1*l^4*v*x*y^2*cos(theta)^4*cos(z)*sin(theta) - 4*a0*a1*l^4*r^2*v*y*cos(theta)^4*sin(theta)*sin(z) + 4*a0*a1*l^4*v*x^2*y*cos(theta)^4*sin(theta)*sin(z) - 8*a1*a2*l^3*v^3*x^2*cos(theta)^3*cos(z)*sin(theta)^2*sin(z) + 8*a1*a2*l^3*v^3*y^2*cos(theta)^3*cos(z)*sin(theta)^2*sin(z) - 8*a2^2*l^2*v^4*x*y*cos(theta)^2*cos(z)*sin(theta)^3*sin(z)))/(8*l^2*v^4*cos(theta)*(y*cos(z) - x*sin(z))^2)];

else
    
       w0 = [0;0;0];
       w1 = w0;
    
end    
    
w_m = w0+d/2*w1; 


if pathType == 1
    alpha = x^2+y^2 - r^2;
else
    a       = 3; b       = 1.05*a;
    alpha = (x^2+y^2+a^2)^2-4*a^2*x^2-b^4; % defines the path
end
if alpha < 1e-2 && Change == 1
    ref = 2*v_ref;
else
    ref = v_ref;
end



u    = -[L0 L1]*[(v-ref);amr]; 

if c == 0  
    w = w_m(1); 
elseif c == 1
    w = w_m(2); 
else
    w = w_m(3); 
end

== matlab function AcermanDynExt/MATLAB Function6 ==
  data: c_old input; c output
function c  = fcn(c_old)

if c_old < 3
    c = c_old+1; 
else 
    c = 0;  
end

== matlab function AcermanDynExt/MATLAB Function7 ==
  data: ref_old input; delta_b input; ref_x1 output; v0 input; ref_x output; m parameter
function [ref_x1,ref_x] = fcn(ref_old, delta_b, v0, m)
delta = delta_b*3; 
a1 = m;
ref_old(2) = 0; 

ref_x1 = ref_old + [delta*v0*a1; v0*a1];

ref_x2 = ref_x1 + [delta*v0*a1; v0*a1];
ref_x = [ref_x1 ref_x2];

== matlab function AcermanDynExt/MATLAB Function8 ==
  data: tnref input; ref output; refType parameter; v_ref parameter
function ref = fcn(tnref,refType,v_ref)

if (refType == 1)
    ref = v_ref;
else
%     ref = tnref(1,2);
        ref = v_ref;
end

== matlab function AcermanDynExt/MATLAB Function10 ==
  data: state input; v input; vsdd input; v_ref input; pathType parameter; r parameter; k0 parameter; l parameter; utn output; utr output; Change parameter; T parameter; refType parameter; k1 parameter
function [utn,utr] = MATLAB_Function5(state, v, vsdd, v_ref,pathType, r, k0, l , Change, T, refType, k1)

x = state(1); y = state(2); theta = state(3); phi = state(4);
eta1 = v; eta2 = vsdd;

if pathType == 1
    D = [ -(y*cos(theta) - x*sin(theta))/(x^2 + y^2), (eta1^2*(x*cos(theta) + y*sin(theta)))/(l*cos(phi)^2*(x^2 + y^2));
            2*x*cos(theta) + 2*y*sin(theta),           (2*eta1^2*(y*cos(theta) - x*sin(theta)))/(l*cos(phi)^2)];
    F  = [  (eta1*(sin(phi)*x^2 - 2*l*cos(phi)*sin(theta)*x + sin(phi)*y^2 + 2*l*cos(phi)*cos(theta)*y)*(eta1^2*l*x^2*cos(phi) - 3*eta1^2*l*y^2*cos(phi) + eta1^2*y^3*cos(theta)*sin(phi) - eta1^2*x^3*sin(phi)*sin(theta) + eta1^2*x^2*y*cos(theta)*sin(phi) - eta1^2*x*y^2*sin(phi)*sin(theta) - 4*eta1^2*l*x^2*cos(phi)*cos(theta)^2 + 4*eta1^2*l*y^2*cos(phi)*cos(theta)^2 + 3*eta2*l*x^3*cos(phi)*cos(theta) + 3*eta2*l*y^3*cos(phi)*sin(theta) + 3*eta2*l*x*y^2*cos(phi)*cos(theta) + 3*eta2*l*x^2*y*cos(phi)*sin(theta) - 8*eta1^2*l*x*y*cos(phi)*cos(theta)*sin(theta)))/(l^2*cos(phi)^2*(x^2 + y^2)^3);
                                                                                                                                                                                                                                                                                                                                           (2*eta1*(3*eta2*l^2*cos(phi)^2*sin(theta)^2 - eta1^2*x*cos(theta)*sin(phi)^2 - eta1^2*y*sin(phi)^2*sin(theta) + 3*eta2*l^2*cos(phi)^2*cos(theta)^2 + 3*eta2*l*y*cos(phi)*cos(theta)*sin(phi) - 3*eta2*l*x*cos(phi)*sin(phi)*sin(theta)))/(l^2*cos(phi)^2)];
else

    D = [ -(y*cos(theta)-x*sin(theta))/(x^2 + y^2),  (eta1^2*(x*cos(theta)+y*sin(theta)))/(cos(phi)^2*(x^2+y^2));
         4*x*cos(theta)*(x^2 + y^2-9)+4*y*sin(theta)*(x^2 + y^2+9),    eta1*(tan(phi)^2+1)*(4*y*eta1*cos(theta)*(x^2 + y^2+9)-4*x*eta1*sin(theta)*(x^2 + y^2-9))];
 
     F  = [ (eta1*(sin(phi)*x^2-2*cos(phi)*sin(theta)*x+sin(phi)*y^2+2*cos(theta)*cos(phi)*y)*(x^2*eta1^2*cos(phi)-3*y^2*eta1^2*cos(phi)-4*x^2*eta1^2*cos(theta)^2*cos(phi)+4*y^2*eta1^2*cos(theta)^2*cos(phi)+3*x^3*eta2*cos(theta)*cos(phi)+3*y^3*eta2*cos(phi)*sin(theta)+y^3*eta1^2*cos(theta)*sin(phi)-x^3*eta1^2*sin(theta)*sin(phi)+x^2*y*eta1^2*cos(theta)*sin(phi)-x*y^2*eta1^2*sin(theta)*sin(phi)+3*x*y^2*eta2*cos(theta)*cos(phi)+3*x^2*y*eta2*cos(phi)*sin(theta)-8*x*y*eta1^2*cos(theta)*cos(phi)*sin(theta)))/(cos(phi)^2*(x^2 + y^2)^3);
       (36*x*eta1^3*cos(theta) + 108*eta1*eta2*cos(phi)^2 - 36*y*eta1^3*sin(theta) - 4*x^3*eta1^3*cos(theta) - 4*y^3*eta1^3*sin(theta) + 4*x^3*eta1^3*cos(theta)*cos(phi)^2 + 4*y^3*eta1^3*cos(phi)^2*sin(theta) - 4*x*y^2*eta1^3*cos(theta) + 12*x^2*eta1*eta2*cos(phi)^2 + 36*y^2*eta1*eta2*cos(phi)^2 - 12*x*y*eta1^3*sin(2*phi) - 4*x^2*y*eta1^3*sin(theta) - 12*x*eta1^3*cos(theta)*cos(phi)^2 - 216*eta1*eta2*cos(theta)^2*cos(phi)^2 + 60*y*eta1^3*cos(phi)^2*sin(theta) + 4*x*y^2*eta1^3*cos(theta)*cos(phi)^2 + 24*x^2*eta1*eta2*cos(theta)^2*cos(phi)^2 - 24*y^2*eta1*eta2*cos(theta)^2*cos(phi)^2 + 4*x^2*y*eta1^3*cos(phi)^2*sin(theta) + 216*eta1^3*cos(theta)*cos(phi)*sin(theta)*sin(phi) + 48*x*y*eta1^3*cos(theta)^2*cos(phi)*sin(phi) + 108*y*eta1*eta2*cos(theta)*cos(phi)*sin(phi) + 108*x*eta1*eta2*cos(phi)*sin(theta)*sin(phi) - 24*x^2*eta1^3*cos(theta)*cos(phi)*sin(theta)*sin(phi) + 24*y^2*eta1^3*cos(theta)*cos(phi)*sin(theta)*sin(phi) + 12*y^3*eta1*eta2*cos(theta)*cos(phi)*sin(phi) - 12*x^3*eta1*eta2*cos(phi)*sin(theta)*sin(phi) + 48*x*y*eta1*eta2*cos(theta)*cos(phi)^2*sin(theta) + 12*x^2*y*eta1*eta2*cos(theta)*cos(phi)*sin(phi) - 12*x*y^2*eta1*eta2*cos(phi)*sin(theta)*sin(phi))/cos(phi)^2];
    
end

  
Di = pinv(D);

if pathType == 1
    alpha = x^2+y^2 - r^2;
    psi1 = x^2+y^2-r^2; %
    psi2 = 2*eta1*(x*cos(theta) + y*sin(theta));
    psi3 = 2*eta1^2*cos(theta)^2 + 2*eta1^2*sin(theta)^2 + eta2*(2*x*cos(theta) + 2*y*sin(theta)) + (2*eta1^2*tan(phi)*(y*cos(theta) - x*sin(theta)))/l;
else
    a       = 3; b       = 1.05*a;
    alpha = (x^2+y^2+a^2)^2-4*a^2*x^2-b^4; % defines the path
    psi1 = (x^2+y^2+a^2)^2-4*a^2*x^2-b^4;
    psi2 = 4*x*eta1*cos(theta)*(x^2 + y^2 - 9) + 4*y*eta1*sin(theta)*(x^2 + y^2 + 9);
    psi3 = eta2*(4*x*cos(theta)*(x^2 + y^2 - 9) + 4*y*sin(theta)*(x^2 + y^2 + 9)) + eta1*cos(theta)*(8*x^2*eta1*cos(theta) + 4*eta1*cos(theta)*(x^2 + y^2 - 9) + 8*x*y*eta1*sin(theta)) + eta1*sin(theta)*(8*y^2*eta1*sin(theta) + 4*eta1*sin(theta)*(x^2 + y^2 + 9) + 8*x*y*eta1*cos(theta)) + eta1*tan(phi)*(4*y*eta1*cos(theta)*(x^2 + y^2 + 9) - 4*x*eta1*sin(theta)*(x^2 + y^2 - 9));
end

if alpha < 1e-2 && Change == 1
    ref = 2*v_ref;
else
    ref = v_ref;
end

z1 = atan2(y,x);
z2 = -(eta1*(y*cos(theta) - x*sin(theta)))/(x^2 + y^2);
z3 = (eta1^2*cos(theta)*(- sin(theta)*x^2 + 2*cos(theta)*x*y + sin(theta)*y^2))/(x^2 + y^2)^2 - (eta2*(y*cos(theta) - x*sin(theta)))/(x^2 + y^2) - (eta1^2*sin(theta)*(cos(theta)*x^2 + 2*sin(theta)*x*y - cos(theta)*y^2))/(x^2 + y^2)^2 + (eta1^2*tan(phi)*(x*cos(theta) + y*sin(theta)))/(x^2 + y^2);
 

delta = T;
psi = [psi1-delta*psi2+delta^2/3*psi3;psi2-delta*psi3;psi3];
zeta = [z1-delta*z2+delta^2/3*z3;z2-delta*z3;z3];

lamda1 = k0; lamda2 = k0;
L0 = -(exp(-T*lamda1) + exp(-T*lamda2) - exp(-T*lamda1)*exp(-T*lamda2) - 1)/T^2;
L1 = -(exp(-T*lamda1) + exp(-T*lamda2) + exp(-T*lamda1)*exp(-T*lamda2) - 3)/(2*T);

usd1 = -k0*(eta1-ref)-k0*eta2;
usd1 =  -L0*(eta1-ref)-L1*eta2;

usd2 =  k1*psi;

u  = Di*([usd1;usd2]-F);
utn = u(1); 
utr = u(2);

== matlab function AcermanDynExt/MATLAB Function9 ==
  data: x output; state input; y output; theta output; emr output; pathType parameter; r parameter; a parameter; b parameter
function [x, y, theta, emr] = fcn(state, pathType, r, a, b)

x = state(1);
y = state(2);
theta = state(3);
if pathType == 1
    emr = x^2+y^2 - r^2;
else
    emr = (x^2+y^2+a^2)^2-4*a^2*x^2-b^4;
    
end

== matlab function AcermanDynExt/MATLAB Function11 ==
  data: x output; state input; y output; theta output
function [x, y, theta] = fcn(state)

x = state(1);
y = state(2);
theta = state(3);
